simulink model "AttitudeDynamics"  (R2017b)
settings: Solver=VariableStepAuto  StartTime=0.0  StopTime=100  FixedStep=1  MaxStep=0.1  RelTol=1e-6  EnableMultiTasking=on
StopFcn:
  | close all
  | 
  | %figure(1)
  | %attitudePlot = animateAttitude(rotmOut, 0.016);
  | %attitudePlot.plotInit;
  | 
  | 
  | responsePlot(Response_data.signals.values, Response_data.time);
values from neighbouring files (symbols this model uses):
  J_sat = [2.5 2.5 2.5]    [AttitudeDynamicsData.m]
  J_sphere = 0.005567928416632    (= 0.00556792841663)    [AttitudeDynamicsData.m]
  T_disturb = ones(1,3) * 0.1E-3    [AttitudeDynamicsData.m]
libraries: SatelliteLibrary x7, simulink x1, mpclib x1
settings Model: Creator=Huib  LastModifiedBy=Laurens
settings DataIOCC: LimitDataPoints=on
settings OptimizationCC: LifeSpan=inf
settings DebuggingCC: AllowSymbolicDim=off  SFUnexpectedBacktrackingDiag=warning  SFNoUnconditionalDefaultTransitionDiag=warning  SFExecutionAtInitializationDiag=none
settings ModelReferenceCC: PropagateSignalLabelsOutOfModel=off
settings CodeAppCC: StateflowObjectComments=on
settings GRTTargetCC: TargetLangStandard=C89/C90 (ANSI)
settings ConfigComp: CovMetricSettings=dw  CovHtmlReporting=on  CovSaveCumulativeToWorkspaceVar=on  CovSaveSingleToWorkspaceVar=on  CovExternalEMLEnable=off

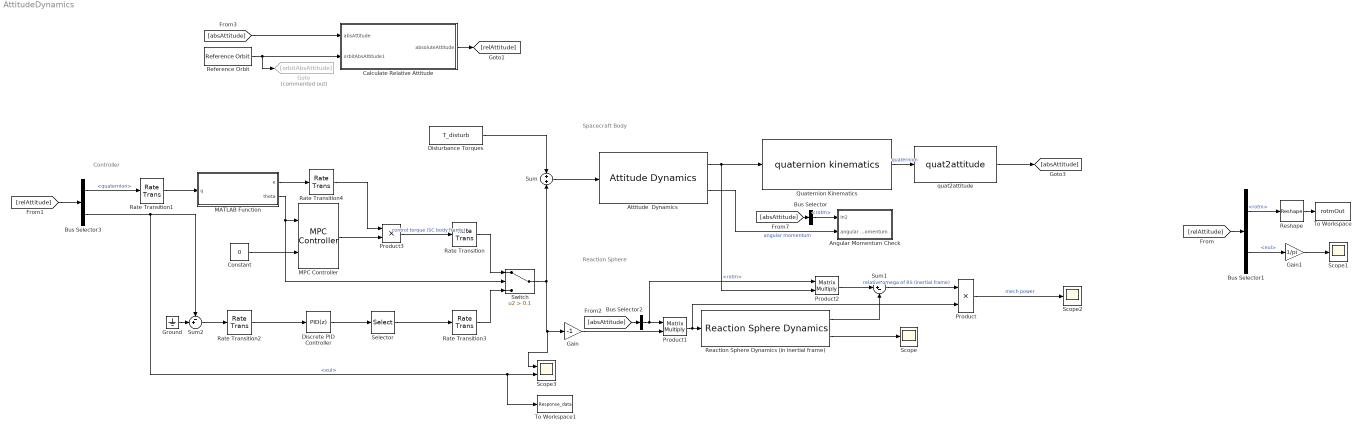
== system AttitudeDynamics ==
  note: Reaction Sphere
  note: Controller
  note: Spacecraft Body
  Angular Momentum Check : Subsystem
  Attitude  Dynamics : SatelliteLibrary/Attitude Dynamics  J11=J_sat(1)  J22=J_sat(2)  J33=J_sat(3)  omega0=w_zero
  Bus Selector : BusSelector  OutputSignals=rotm
  Bus Selector1 : BusSelector  OutputSignals=rotm,eul
  Bus Selector2 : BusSelector  OutputSignals=rotm
  Bus Selector3 : BusSelector  OutputSignals=quaternion,eul
  Calculate Relative Attitude : Subsystem
  Constant : Constant  Value=0
  Discrete PID Controller : simulink/Continuous/PID Controller  Controller=PID  TimeDomain=Discrete-time  SampleTime=-1  IntegratorMethod=Forward Euler  FilterMethod=Forward Euler  Form=Parallel  UseFilter=on  ControllerParametersSource=internal  P=0.0216487535462019  I=0.000210079243058548  D=0.543508472205106  N=1.14439525064094  InitialConditionSource=internal  InitialConditionForIntegrator=0  InitialConditionForFilter=0  ExternalReset=none  LimitOutput=off  UpperSaturationLimit=inf  LowerSaturationLimit=-inf  LinearizeAsGain=off  AntiWindupMode=none  Kb=1  TrackingMode=off  Kt=1  PParamMin=[]  PParamMax=[]  IParamMin=[]  IParamMax=[]  DParamMin=[]  DParamMax=[]  NParamMin=[]  NParamMax=[]  KbParamMin=[]  KbParamMax=[]  KtParamMin=[]  KtParamMax=[]  POutMin=[]  POutMax=[]  IOutMin=[]  IOutMax=[]  DOutMin=[]  DOutMax=[]  NOutMin=[]  NOutMax=[]  KbOutMin=[]  KbOutMax=[]  KtOutMin=[]  KtOutMax=[]  IntegratorOutMin=[]  IntegratorOutMax=[]  FilterOutMin=[]  FilterOutMax=[]  SumOutMin=[]  SumOutMax=[]  SumI1OutMin=[]  SumI1OutMax=[]  SumI2OutMin=[]  SumI2OutMax=[]  SumI3OutMin=[]  SumI3OutMax=[]  SumDOutMin=[]  SumDOutMax=[]  SaturationOutMin=[]  SaturationOutMax=[]  IntegratorContinuousStateAttributes=''  IntegratorStateMustResolveToSignalObject=off  IntegratorRTWStateStorageClass=Auto  FilterContinuousStateAttributes=''  FilterStateMustResolveToSignalObject=off  FilterRTWStateStorageClass=Auto  DifferentiatorICPrevScaledInput=0  DifferentiatorOutMin=[]  DifferentiatorOutMax=[]  InitialConditionSetting=State (most efficient)  FilterDiffOutCoefMin=[]  FilterDiffOutCoefMax=[]  SumDenOutMin=[]  SumDenOutMax=[]  SumNumOutMin=[]  SumNumOutMax=[]  ReciprocalOutMin=[]  ReciprocalOutMax=[]  DivideOutMin=[]  DivideOutMax=[]  TunerSelectOption=Transfer Function Based (PID Tuner App)
  Disturbance Torques : Constant  Value=T_disturb
  Gain : Gain  Gain=-1
  Gain1 : Gain  Gain=1/pi
  Goto : Goto  Commented=on  GotoTag=orbitAbsAttitude
  Ground : Ground
  MATLAB Function : MATLAB Function  TreatAsAtomicUnit=on
  MPC Controller : mpclib/MPC Controller  SCDEnableBlockLinearizationSpecification=on  mpcobj=mpc1  is_multiple=0  enable_value=0  return_u0=off  ref_from_ws=off  ref_signal_name=[]  ref_preview=off  md_from_ws=off  md_signal_name=[]  md_preview=off  from_project=off  project_file=MPCtask.mat  md_inport=off  mv_inport=off  cost_outport=off  return_sequence=off  return_qpstatus=off  return_state=off  state_inport=off  lims_inport=off  cc_inport=off  ywt_inport=off  is_designfromscratch=0  uwt_inport=off  duwt_inport=off  rhoeps_inport=off  uref_inport=off  n_ts=1  n_p=20  n_mv=1  n_md=0  n_ud=0  n_mo=1  n_uo=0  BlockDataType=double  SampleTimeInherited=off  switch_inport=off
  Product : Product
  Product1 : Product  Multiplication=Matrix(*)
  Product2 : Product  Multiplication=Matrix(*)
  Product3 : Product
  Quaternion Kinematics : SatelliteLibrary/quaternion kinematics  q_0=q_zero
  Rate Transition : RateTransition
  Rate Transition1 : RateTransition  OutPortSampleTime=0.1
  Rate Transition2 : RateTransition  OutPortSampleTime=0.1
  Rate Transition3 : RateTransition
  Rate Transition4 : RateTransition  OutPortSampleTime=1
  Reaction Sphere Dynamics (in inertial frame) : SatelliteLibrary/Reaction Sphere Dynamics  J=J_sphere  omega0=[0 0 0]
  Reference Orbit : SatelliteLibrary/Reference Orbit  orbitAltitude=700  gravParam=398600.4418  planetRadius=6371
  Reshape : Reshape  OutputDimensions=[9,1]
  Scope : Scope
  Scope1 : Scope
  Scope2 : Scope
  Scope3 : Scope  NumInputPorts=2
  Selector : Selector  InputPortWidth=3  IndexOptions=Index vector (dialog)  Indices=[3 2 1]  OutputSizes=1
  Sum : Sum  Inputs=+|+
  Sum1 : Sum  Inputs=|+-
  Sum2 : Sum  Inputs=-+|
  Switch : Switch  Criteria=u2 > Threshold  Threshold=0.1
  To Workspace : ToWorkspace  VariableName=rotmOut  SaveFormat=Timeseries  SampleTime=-1
  To Workspace1 : ToWorkspace  VariableName=Response_data  SaveFormat=Structure With Time  SampleTime=-1
      settings: Decimation=2
  quat2attitude : SatelliteLibrary/quat2attitude
  wires:
  Attitude  Dynamics/1 -> Product2/2, Quaternion Kinematics/1
  Quaternion Kinematics/1 -> quat2attitude/1  "quaternion"
  Sum/1 -> Attitude  Dynamics/1
  Reshape/1 -> To Workspace/1
  Product1/1 -> Product/2, Reaction Sphere Dynamics (in inertial frame)/1
  Product3/1 -> Rate Transition/1  "control torque (SC body frame)"
  Gain/1 -> Product1/2
  Attitude  Dynamics/2 -> Angular Momentum Check/2(angular momentum)  "angular momentum"
  Bus Selector1/1 -> Reshape/1  "<rotm>"
  Bus Selector/1 -> Angular Momentum Check/1(In2)  "<rotm>"
  Bus Selector2/1 -> Product2/1, Product1/1  "<rotm>"
  Reaction Sphere Dynamics (in inertial frame)/1 -> Sum1/2
  Reaction Sphere Dynamics (in inertial frame)/2 -> Scope/1
  Gain1/1 -> Scope1/1
  Product2/1 -> Sum1/1
  Sum1/1 -> Product/1  "relative omega of RS (inertial frame)"
  Product/1 -> Scope2/1  "mech power"
  [absAttitude] -> Bus Selector/1
  [absAttitude] -> Bus Selector2/1
  [relAttitude] -> Bus Selector1/1
  Bus Selector1/2 -> Gain1/1  "<eul>"
  [absAttitude] -> Calculate Relative Attitude/1(absAttitude)
  Calculate Relative Attitude/1(absoluteAttitude) -> [relAttitude]
  quat2attitude/1 -> [absAttitude]
  Reference Orbit/1 -> Goto/1, Calculate Relative Attitude/2(orbitAbsAttitude1)
  Bus Selector3/1 -> Rate Transition1/1  "<quaternion>"
  [relAttitude] -> Bus Selector3/1
  MATLAB Function/2(theta) -> Switch/2, MPC Controller/1
  MPC Controller/1 -> Product3/2
  Constant/1 -> MPC Controller/2
  Disturbance Torques/1 -> Sum/1
  Switch/1 -> Sum/2, Scope3/1, Gain/1
  MATLAB Function/1(e) -> Rate Transition4/1
  Rate Transition1/1 -> MATLAB Function/1(q)
  Bus Selector3/2 -> To Workspace1/1, Scope3/2, Sum2/1  "<eul>"
  Ground/1 -> Sum2/2
  Sum2/1 -> Rate Transition2/1
  Rate Transition2/1 -> Discrete PID Controller/1
  Discrete PID Controller/1 -> Selector/1
  Rate Transition/1 -> Switch/1
  Rate Transition3/1 -> Switch/3
  Rate Transition4/1 -> Product3/1
  Selector/1 -> Rate Transition3/1

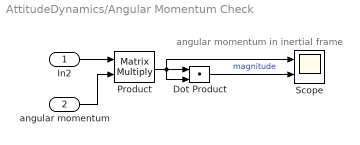
== system AttitudeDynamics/Angular Momentum Check ==
  note: angular momentum in inertial frame
  In2 : Inport
  angular momentum : Inport  Port=2
  Dot Product : DotProduct  InputSameDT=on  OutDataTypeStr=Inherit: Inherit via internal rule
  Product : Product  Multiplication=Matrix(*)
  Scope : Scope  NumInputPorts=2
  wires:
  angular momentum/1 -> Product/2
  Product/1 -> Scope/1, Dot Product/2, Dot Product/1
  Dot Product/1 -> Scope/2  "magnitude"
  In2/1 -> Product/1

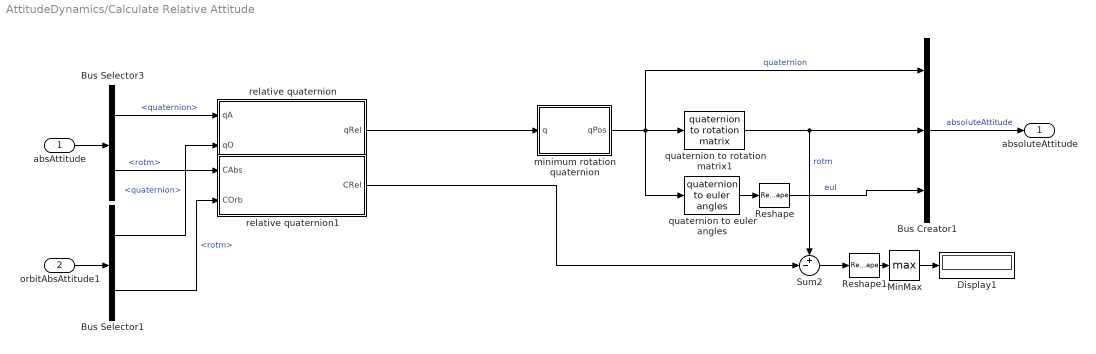
== system AttitudeDynamics/Calculate Relative Attitude ==
  absAttitude : Inport
  orbitAbsAttitude1 : Inport  Port=2
  Bus Creator1 : BusCreator  Inputs=3
  Bus Selector1 : BusSelector  OutputSignals=quaternion,rotm
  Bus Selector3 : BusSelector  OutputSignals=quaternion,rotm
  Display1 : Display
  MinMax : MinMax  Function=max  ZeroCross=off
  Reshape : Reshape
  Reshape1 : Reshape
  Sum2 : Sum  Inputs=+-|
  minimum rotation quaternion : MATLAB Function  TreatAsAtomicUnit=on
  quaternion to euler angles : SatelliteLibrary/quaternion to euler angles
  quaternion to rotation matrix1 : SatelliteLibrary/quaternion to rotation matrix
  relative quaternion : MATLAB Function  TreatAsAtomicUnit=on
  relative quaternion1 : MATLAB Function  TreatAsAtomicUnit=on
  absoluteAttitude : Outport
  wires:
  Bus Selector1/1 -> relative quaternion/2(qO)  "<quaternion>"
  Bus Selector3/2 -> relative quaternion1/1(CAbs)  "<rotm>"
  Reshape1/1 -> MinMax/1
  MinMax/1 -> Display1/1
  relative quaternion1/1(CRel) -> Sum2/2
  quaternion to rotation matrix1/1 -> Sum2/1, Bus Creator1/2  "rotm"
  Bus Creator1/1 -> absoluteAttitude/1  "absoluteAttitude"
  minimum rotation quaternion/1(qPos) -> Bus Creator1/1, quaternion to euler angles/1, quaternion to rotation matrix1/1  "quaternion"
  quaternion to euler angles/1 -> Reshape/1
  Bus Selector3/1 -> relative quaternion/1(qA)  "<quaternion>"
  Sum2/1 -> Reshape1/1
  relative quaternion/1(qRel) -> minimum rotation quaternion/1(q)
  Bus Selector1/2 -> relative quaternion1/2(COrb)  "<rotm>"
  absAttitude/1 -> Bus Selector3/1
  orbitAbsAttitude1/1 -> Bus Selector1/1
  Reshape/1 -> Bus Creator1/3  "eul"

== matlab function AttitudeDynamics/Calculate Relative Attitude/minimum rotation quaternion ==
  data: q input; qPos output
function qPos = minRotation(q)
    % converts quaternion to form of smalest angle (last element always <0, 1])
    if q(4) < 0
        qPos = -q;
    else
        qPos = q;
    end
end

== matlab function AttitudeDynamics/MATLAB Function ==
  data: q input; e output; theta output
function [e, theta] = quat2axisAngle(q)
%#codegen
theta = 2 * acos(q(4));
if theta == 0
    e = zeros(3,1);
else
    e = q(1:3) / sin(theta/2);
end

== matlab function AttitudeDynamics/Calculate Relative Attitude/relative quaternion1 ==
  data: CAbs input; COrb input; CRel output
function CRel = rotmatRelative(...
    CAbs, ... absolute rotation matrix orientation (in inertial reference frame)
    COrb  ... orbital frame rotation matrix orientation
    )

CRel = COrb \ CAbs;
end

== matlab function AttitudeDynamics/Calculate Relative Attitude/relative quaternion ==
  data: qA input; qO input; qRel output
function qRel = quatRelative(...
    qA, ... absolute quaternion orientation (in inertial reference frame)
    qO  ... orbital frame quaternion orientation
    )
% Calculate the error quaternion
% q_... are standard quaternions with the vector part at the start

qOinv = [-qO(1:3); qO(4)];
qAmatrix = [ qA(4)  qA(3) -qA(2)  qA(1);...
            -qA(3)  qA(4)  qA(1)  qA(2);...
             qA(2) -qA(1)  qA(4)  qA(3);...
            -qA(1) -qA(2) -qA(3)  qA(4)];
qRel = qAmatrix * qOinv;
end
